simulink model "SEDCmotor"  (R2018a)
settings: Solver=VariableStepAuto  StartTime=0.0  StopTime=15  RelTol=1e-3
values from neighbouring files (symbols this model uses):
  Bm = 0.00000604    (= 6.04e-06)    [PMDCparameters.m]    (also in SEDCparameters.m = 1.074e-06; SeriseDCparameters.m = 0.0025; ShuntDCparameters.m = 1.074e-06)
  J = 0.00000161    (= 1.61e-06)    [PMDCparameters.m]    (also in SEDCparameters.m = 0.21; SeriseDCparameters.m = 0.02365; ShuntDCparameters.m = 0.21)
  LAA = 0.12    [PMDCparameters.m]    (also in SEDCparameters.m = 0.01; SeriseDCparameters.m; ShuntDCparameters.m = 0.01)
  LAF = 0.004    [SEDCparameters.m]    (also in SeriseDCparameters.m = 0.0675; ShuntDCparameters.m)
  LFF = 0.167    [SEDCparameters.m]    (also in SeriseDCparameters.m = 0.03; ShuntDCparameters.m)
  ra = 7    [PMDCparameters.m]    (also in SEDCparameters.m = 0.013; SeriseDCparameters.m = 1.5; ShuntDCparameters.m = 0.013)
  rf = 1.43    [SEDCparameters.m]    (also in SeriseDCparameters.m = 0.7; ShuntDCparameters.m)
  Tl = 0.003    [PMDCparameters.m]    (also in SEDCparameters.m = 2.493; SeriseDCparameters.m = 10; ShuntDCparameters.m = 2.493)
  Va = 6    [PMDCparameters.m]    (also in SEDCparameters.m = 24; SeriseDCparameters.m = 100; ShuntDCparameters.m = 24)
  Vf = 12    [SEDCparameters.m]    (also in SeriseDCparameters.m = 100; ShuntDCparameters.m)
libraries: fl_lib x17, nesl_utility x12, powerlib x4
settings Model: Creator=Noor  LastModifiedBy=Noor

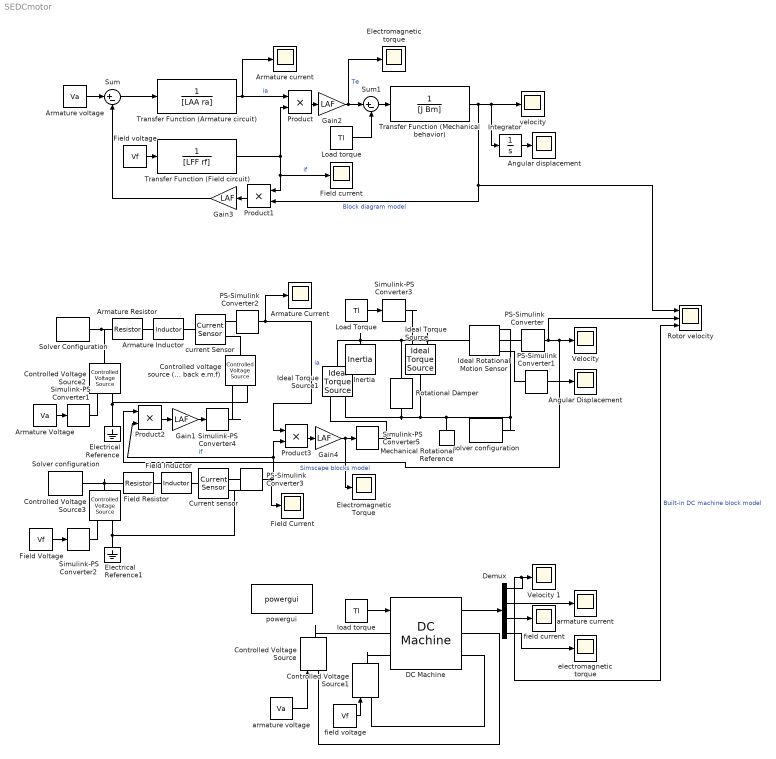
== system SEDCmotor ==
  " Ideal Torque Source" : fl_lib/Mechanical/Mechanical Sources/Ideal Torque Source
  Angular Displacement : Scope
  Angular displacement : Scope
  Armature Inductor : fl_lib/Electrical/Electrical Elements/Inductor  l=LAA H  r=0 Ohm  g=0 1/Ohm  i_specify=off  i_priority=None  i=0 A  i_nominal_specify=off  i_nominal_unit=A  i_nominal_value=1  v_specify=off  v_priority=None  v=0 V  v_nominal_specify=off  v_nominal_unit=V  v_nominal_value=1  i_L_specify=off  i_L_priority=High  i_L=0 A  i_L_nominal_specify=off  i_L_nominal_unit=A  i_L_nominal_value=1
  Armature Resistor : fl_lib/Electrical/Electrical Elements/Resistor  R=ra Ohm  i_specify=off  i_priority=None  i=0 A  i_nominal_specify=off  i_nominal_unit=A  i_nominal_value=1  v_specify=off  v_priority=None  v=0 V  v_nominal_specify=off  v_nominal_unit=V  v_nominal_value=1
  Armature Current : Scope
  Armature Voltage : Constant  Value=Va
  Armature current : Scope
  Armature voltage : Constant  Value=Va
  Controlled voltage source (i.e. back e.m.f) : fl_lib/Electrical/Electrical Sources/Controlled Voltage Source
  Controlled Voltage Source2 : fl_lib/Electrical/Electrical Sources/Controlled Voltage Source
  Controlled Voltage Source3 : fl_lib/Electrical/Electrical Sources/Controlled Voltage Source
  Controlled Voltage Source : powerlib/Electrical Sources/Controlled Voltage Source  Initialize=on  Source_Type=AC  Amplitude=0  Phase=0  Frequency=0  Measurements=None
  Controlled Voltage Source1 : powerlib/Electrical Sources/Controlled Voltage Source  Initialize=on  Source_Type=AC  Amplitude=0  Phase=0  Frequency=0  Measurements=None
  Current sensor : fl_lib/Electrical/Electrical Sensors/Current Sensor
  DC Machine : powerlib/Machines/DC Machine  PresetModel=No  MechanicalLoad=Torque TL  FieldType=Wound  ShowDetailedParameters=on  MeasurementBus=off  RLa=[ra LAA]  RLf=[rf LFF]  Laf=LAF  MachineConstant=Torque constant (N.m/A)  Ke=1.8  Kt=1.8  J=J  Bm=Bm  Tf=0  w0=0  Ifinit=0  TsPowergui=0  TsBlock=-1
  Demux : Demux
  Electrical Reference : fl_lib/Electrical/Electrical Elements/Electrical Reference
  Electrical Reference1 : fl_lib/Electrical/Electrical Elements/Electrical Reference
  Electromagnetic Torque : Scope
  "Electromagnetic torque " : Scope
  Field Inductor : fl_lib/Electrical/Electrical Elements/Inductor  l=LFF H  r=0 Ohm  g=0 1/Ohm  i_specify=off  i_priority=None  i=0 A  i_nominal_specify=off  i_nominal_unit=A  i_nominal_value=1  v_specify=off  v_priority=None  v=0 V  v_nominal_specify=off  v_nominal_unit=V  v_nominal_value=1  i_L_specify=off  i_L_priority=High  i_L=0 A  i_L_nominal_specify=off  i_L_nominal_unit=A  i_L_nominal_value=1
  Field Resistor : fl_lib/Electrical/Electrical Elements/Resistor  R=rf Ohm  i_specify=off  i_priority=None  i=0 A  i_nominal_specify=off  i_nominal_unit=A  i_nominal_value=1  v_specify=off  v_priority=None  v=0 V  v_nominal_specify=off  v_nominal_unit=V  v_nominal_value=1
  Field Current : Scope
  Field Voltage : Constant  Value=Vf
  Field current : Scope
  Field voltage : Constant  Value=Vf
  Gain{1..4} (4 alike) : Gain  Gain=LAF
  Ideal Rotational Motion Sensor : fl_lib/Mechanical/Mechanical Sensors/Ideal Rotational Motion Sensor  offset=0 rev
  Ideal Torque Source1 : fl_lib/Mechanical/Mechanical Sources/Ideal Torque Source
  "Inertia " : fl_lib/Mechanical/Rotational Elements/Inertia  inertia=J kg*m^2  w_specify=off  w_priority=High  w=0 rad/s  w_nominal_specify=off  w_nominal_unit=rad/s  w_nominal_value=1  t_specify=off  t_priority=None  t=0 N*m  t_nominal_specify=off  t_nominal_unit=N*m  t_nominal_value=1
  Integrator : Integrator
  Load Torque : Constant  Value=Tl
  Load torque : Constant  Value=Tl
  Mechanical Rotational Reference : fl_lib/Mechanical/Rotational Elements/Mechanical Rotational Reference
  PS-Simulink Converter{,1..3} (4 alike) : nesl_utility/PS-Simulink Converter  PhysicalDomain=network_engine_domain  SubClassName=ps_output  LeftPortType=input  RightPortType=output  PseudoPeriodic=off  Frequencies=[]  Unit=1  AffineConversion=off
  Product{,1..3} (4 alike) : Product
  "Rotational Damper  " : fl_lib/Mechanical/Rotational Elements/Rotational Damper  D=Bm N*m/(rad/s)  w_specify=off  w_priority=None  w=0 rad/s  w_nominal_specify=off  w_nominal_unit=rad/s  w_nominal_value=1  t_specify=off  t_priority=None  t=0 N*m  t_nominal_specify=off  t_nominal_unit=N*m  t_nominal_value=1
  Rotor velocity : Scope  NumInputPorts=3
  Simulink-PS Converter{1..5} (5 alike) : nesl_utility/Simulink-PS Converter  PhysicalDomain=network_engine_domain  SubClassName=ps_input  LeftPortType=input  RightPortType=output  PseudoPeriodic=off  Frequencies=[]  NoiseDistribution=none  NoiseParameters=[]  Unit=1  AffineConversion=off  FilteringAndDerivatives=provide  SimscapeFilterOrder=1  InputFilterTimeConstant=0.001  UdotUserProvided=0
  Solver configuration : nesl_utility/Solver Configuration  PhysicalDomain=network_engine_domain  SubClassName=solver  LeftPortType=input  RightPortType=generic  Tones=[]  Harmonics=[]  SimulateNoise=off  Profile=off  UseLocalSampling=off  EnableSwitchedLinearOptims=on  FrequencyDomain=off  UseCCode=off  RelTol=0.001  AbsTol=1e-06  MinStep=1e-09  ToWorkspace=off  RevertToSquareIcSolve=off  NumHomotopyIterations=100  PhasorMode=off  PhasorModeNumHarmonics=1  DoDC=off  ResidualTolerance=1e-09  UseLocalSolver=off  LocalSolverChoice=NE_BACKWARD_EULER_ADVANCER  LocalSolverSampleTime=0.001  DoFixedCost=off  MaxNonlinIter=3  MaxModeIter=2  LinearAlgebra=Sparse  EquationFormulation=NE_TIME_EF  DelaysMemoryBudget=1024  AutomaticFiltering=on  FilteringTimeConstant=0.001
  Solver Configuration : nesl_utility/Solver Configuration  PhysicalDomain=network_engine_domain  SubClassName=solver  LeftPortType=input  RightPortType=generic  Tones=[]  Harmonics=[]  SimulateNoise=off  Profile=off  UseLocalSampling=off  EnableSwitchedLinearOptims=on  FrequencyDomain=off  UseCCode=off  RelTol=0.001  AbsTol=1e-06  MinStep=1e-09  ToWorkspace=off  RevertToSquareIcSolve=off  NumHomotopyIterations=100  PhasorMode=off  PhasorModeNumHarmonics=1  DoDC=off  ResidualTolerance=1e-09  UseLocalSolver=off  LocalSolverChoice=NE_BACKWARD_EULER_ADVANCER  LocalSolverSampleTime=0.001  DoFixedCost=off  MaxNonlinIter=3  MaxModeIter=2  LinearAlgebra=Sparse  EquationFormulation=NE_TIME_EF  DelaysMemoryBudget=1024  AutomaticFiltering=on  FilteringTimeConstant=0.001
  Sum : Sum  Inputs=|+-
  Sum1 : Sum  Inputs=|+-
  Transfer Function (Armature circuit) : TransferFcn  Denominator=[LAA ra]
  Transfer Function (Field circuit) : TransferFcn  Denominator=[LFF rf]
  Transfer Function (Mechanical behavior) : TransferFcn  Denominator=[J Bm]
  Velocity : Scope
  Velocity 1 : Scope
  armature current : Scope
  armature voltage : Constant  Value=Va
  "current Sensor " : fl_lib/Electrical/Electrical Sensors/Current Sensor
  "electromagnetic torque " : Scope
  field current : Scope
  field voltage : Constant  Value=Vf
  load torque : Constant  Value=Tl
  powergui : powerlib/powergui  Priority=1  SimulationMode=Continuous  SampleTime=50e-6  frequency=60  Iterations=50  frequencyindice=0  Pbase=100e6  ErrMax=1e-4  UnitsV=kV  UnitsW=MW  buscounter=0  FunctionMessages=off  echomessages=off  EnableUseOfTLC=off  CurrentSourceSwitches=off  DisableSnubberDevices=off  DisableRonSwitches=off  DisableVfSwitches=off  DisplayEquations=off  SolverType=Tustin/Backward Euler (TBE)  Interpol=off  ExternalGateDelay=off  methode=off  Ts=100  x0status=blocks  SPID=on  SwTol=0  HookPort=off  RestoreLinks=warning  ResistiveCurrentMeasurement=off  Frange=[0:2:500]  Ylog=off  Xlog=on  ShowGrid=off  save=off  variable=ZData  structure=0  ZoomFFT=off  StartTime=0.0  cycles=1  DisplayStyle=1  fundamental=60  FreqAxis=off  MaxFrequency=1000  frequencyindicesteady=1  RmsSteady=1  display=off
  solver configuration : nesl_utility/Solver Configuration  PhysicalDomain=network_engine_domain  SubClassName=solver  LeftPortType=input  RightPortType=generic  Tones=[]  Harmonics=[]  SimulateNoise=off  Profile=off  UseLocalSampling=off  EnableSwitchedLinearOptims=on  FrequencyDomain=off  UseCCode=off  RelTol=0.001  AbsTol=1e-06  MinStep=1e-09  ToWorkspace=off  RevertToSquareIcSolve=off  NumHomotopyIterations=100  PhasorMode=off  PhasorModeNumHarmonics=1  DoDC=off  ResidualTolerance=1e-09  UseLocalSolver=off  LocalSolverChoice=NE_BACKWARD_EULER_ADVANCER  LocalSolverSampleTime=0.001  DoFixedCost=off  MaxNonlinIter=3  MaxModeIter=2  LinearAlgebra=Sparse  EquationFormulation=NE_TIME_EF  DelaysMemoryBudget=1024  AutomaticFiltering=on  FilteringTimeConstant=0.001
  velocity : Scope
  wires:
  Transfer Function (Armature circuit)/1 -> Armature current/1, Product/1  "ia"
  Sum/1 -> Transfer Function (Armature circuit)/1
  Sum1/1 -> Transfer Function (Mechanical behavior)/1
  Gain3/1 -> Sum/2
  Armature voltage/1 -> Sum/1
  Field voltage/1 -> Transfer Function (Field circuit)/1
  Product/1 -> Gain2/1
  Transfer Function (Field circuit)/1 -> Product1/1, Field current/1, Product/2  "if"
  Product1/1 -> Gain3/1
  Transfer Function (Mechanical behavior)/1 -> Rotor velocity/1, Product1/2, Integrator/1, velocity/1  "Block diagram model"
  Gain2/1 -> "Electromagnetic torque "/1, Sum1/1  "Te"
  Load torque/1 -> Sum1/2
  DC Machine/1 -> Demux/1
  PS-Simulink Converter3/1 -> Field Current/1, Product3/2, Product2/2  "if"
  PS-Simulink Converter2/1 -> Armature Current/1, Product3/1  "ia"
  Gain1/1 -> Simulink-PS Converter4/1
  Product2/1 -> Gain1/1
  Product3/1 -> Gain4/1
  Load Torque/1 -> Simulink-PS Converter3/1
  Field Voltage/1 -> Simulink-PS Converter2/1
  Armature Voltage/1 -> Simulink-PS Converter1/1
  field voltage/1 -> Controlled Voltage Source1/1
  armature voltage/1 -> Controlled Voltage Source/1
  load torque/1 -> DC Machine/1
  Demux/1 -> Rotor velocity/3, Velocity 1/1  "Built-in DC machine block model"
  PS-Simulink Converter/1 -> Rotor velocity/2, Product2/1, Velocity/1  "Simscape blocks model"
  Demux/4 -> "electromagnetic torque "/1
  Demux/2 -> armature current/1
  Demux/3 -> field current/1
  Gain4/1 -> Electromagnetic Torque/1, Simulink-PS Converter5/1
  Integrator/1 -> Angular displacement/1
  PS-Simulink Converter1/1 -> Angular Displacement/1
  connections:
  Controlled Voltage Source/RConn1 -- DC Machine/LConn1
  Controlled Voltage Source/LConn1 -- DC Machine/RConn1
  Controlled Voltage Source1/RConn1 -- DC Machine/LConn2
  Controlled Voltage Source1/LConn1 -- DC Machine/RConn2
  Solver Configuration/RConn1 -- Controlled Voltage Source2/LConn1 -- Armature Resistor/LConn1
  Controlled Voltage Source2/RConn2 -- Electrical Reference/LConn1 -- Controlled voltage source (i.e. back e.m.f)/RConn2
  "Rotational Damper  "/RConn1 -- Ideal Rotational Motion Sensor/RConn1 -- solver configuration/RConn1 -- Mechanical Rotational Reference/LConn1 -- " Ideal Torque Source"/LConn1 -- Ideal Torque Source1/RConn2
  "current Sensor "/LConn1 -- Armature Inductor/RConn1
  PS-Simulink Converter/LConn1 -- Ideal Rotational Motion Sensor/RConn2
  PS-Simulink Converter2/LConn1 -- "current Sensor "/RConn1
  Controlled Voltage Source2/RConn1 -- Simulink-PS Converter1/RConn1
  Armature Inductor/LConn1 -- Armature Resistor/RConn1
  Solver configuration/RConn1 -- Controlled Voltage Source3/LConn1 -- Field Resistor/LConn1
  Electrical Reference1/LConn1 -- Current sensor/RConn2 -- Controlled Voltage Source3/RConn2
  Field Inductor/LConn1 -- Field Resistor/RConn1
  Current sensor/LConn1 -- Field Inductor/RConn1
  Controlled Voltage Source3/RConn1 -- Simulink-PS Converter2/RConn1
  PS-Simulink Converter3/LConn1 -- Current sensor/RConn1
  Simulink-PS Converter3/RConn1 -- " Ideal Torque Source"/RConn1
  Simulink-PS Converter4/RConn1 -- Controlled voltage source (i.e. back e.m.f)/RConn1
  Simulink-PS Converter5/RConn1 -- Ideal Torque Source1/RConn1
  Controlled voltage source (i.e. back e.m.f)/LConn1 -- "current Sensor "/RConn2
  Ideal Torque Source1/LConn1 -- Ideal Rotational Motion Sensor/LConn1 -- " Ideal Torque Source"/RConn2 -- "Rotational Damper  "/LConn1 -- "Inertia "/LConn1
  PS-Simulink Converter1/LConn1 -- Ideal Rotational Motion Sensor/RConn3
